simulink model "L1_1"  (R2017b)
settings: Solver=ode4  StartTime=0.0  StopTime=30  FixedStep=0.01  RelTol=1e-3
settings Model: Creator=tutuc  LastModifiedBy=tutuc

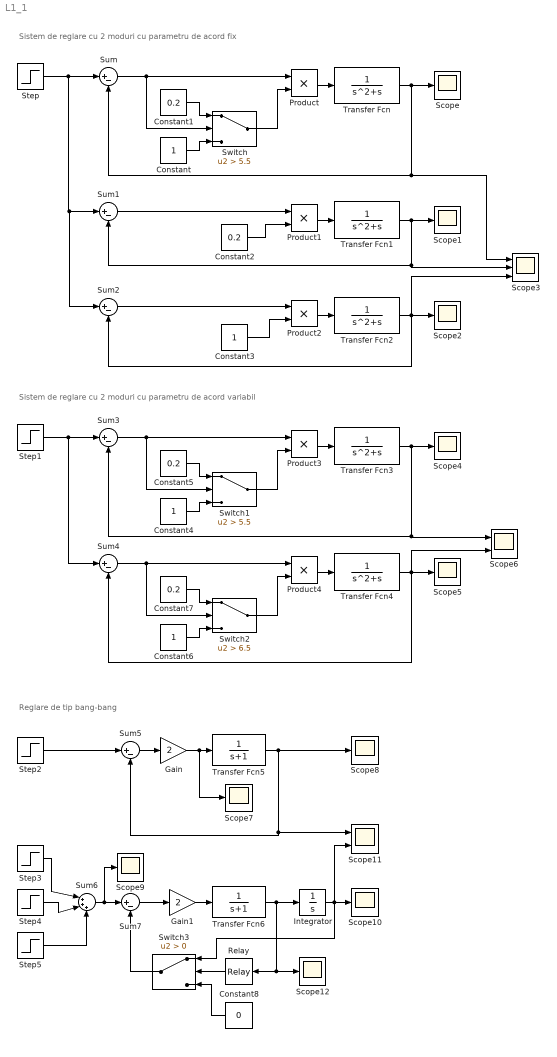
== system L1_1 ==
  note: Sistem de reglare cu 2 moduri cu parametru de acord fix
  note: Sistem de reglare cu 2 moduri cu parametru de acord variabil
  note: Reglare de tip bang-bang
  Constant{,3..4,6} (4 alike) : Constant
  Constant{1..2,5,7} (4 alike) : Constant  Value=0.2
  Constant8 : Constant  Value=0
  Gain : Gain  Gain=2
  Gain1 : Gain  Gain=2
  Integrator : Integrator
  Product{,1..4} (5 alike) : Product
  Relay : Relay  OnSwitchValue=3.1032  OffSwitchValue=-3.1032
  Scope{,1..2,4..5,7..10,12} (10 alike) : Scope
  Scope11 : Scope  NumInputPorts=2
  Scope3 : Scope  NumInputPorts=3
  Scope6 : Scope  NumInputPorts=2
  Step{,1..3} (4 alike) : Step  Time=0  After=10  SampleTime=0
  Step4 : Step  Time=1.35  After=-15  SampleTime=0
  Step5 : Step  Time=1.5  After=5  SampleTime=0
  Sum{,1..5,7} (7 alike) : Sum  Inputs=|+-
  Sum6 : Sum  Inputs=|+++
  Switch : Switch  Criteria=u2 > Threshold  Threshold=5.5
  Switch1 : Switch  Criteria=u2 > Threshold  Threshold=5.5
  Switch2 : Switch  Criteria=u2 > Threshold  Threshold=6.5
  Switch3 : Switch  Criteria=u2 > Threshold
  Transfer Fcn{,1..4} (5 alike) : TransferFcn  Denominator=[1 1 0]
  Transfer Fcn5 : TransferFcn  Denominator=[1 1]
  Transfer Fcn6 : TransferFcn  Denominator=[1 1]
  wires:
  Sum/1 -> Switch/2, Product/1
  Switch/1 -> Product/2
  Step/1 -> Sum2/1, Sum1/1, Sum/1
  Product/1 -> Transfer Fcn/1
  Transfer Fcn/1 -> Scope/1, Sum/2, Scope3/1
  Sum1/1 -> Product1/1
  Constant2/1 -> Product1/2
  Product1/1 -> Transfer Fcn1/1
  Transfer Fcn1/1 -> Scope1/1, Scope3/2, Sum1/2
  Sum2/1 -> Product2/1
  Constant3/1 -> Product2/2
  Product2/1 -> Transfer Fcn2/1
  Transfer Fcn2/1 -> Scope3/3, Scope2/1, Sum2/2
  Constant1/1 -> Switch/1
  Constant/1 -> Switch/3
  Constant4/1 -> Switch1/3
  Constant5/1 -> Switch1/1
  Transfer Fcn3/1 -> Scope6/1, Sum3/2, Scope4/1
  Product3/1 -> Transfer Fcn3/1
  Switch1/1 -> Product3/2
  Sum3/1 -> Product3/1, Switch1/2
  Sum4/1 -> Switch2/2, Product4/1
  Switch2/1 -> Product4/2
  Step1/1 -> Sum3/1, Sum4/1
  Product4/1 -> Transfer Fcn4/1
  Transfer Fcn4/1 -> Scope6/2, Scope5/1, Sum4/2
  Constant7/1 -> Switch2/1
  Constant6/1 -> Switch2/3
  Relay/1 -> Switch3/2
  Gain/1 -> Scope7/1, Transfer Fcn5/1
  Sum7/1 -> Gain1/1
  Switch3/1 -> Sum7/2
  Constant8/1 -> Switch3/3
  Transfer Fcn6/1 -> Scope12/1, Relay/1, Integrator/1
  Step2/1 -> Sum5/1
  Gain1/1 -> Transfer Fcn6/1
  Sum5/1 -> Gain/1
  Step5/1 -> Sum6/3
  Step4/1 -> Sum6/2
  Integrator/1 -> Switch3/1, Scope11/2, Scope10/1
  Step3/1 -> Sum6/1
  Transfer Fcn5/1 -> Sum5/2, Scope11/1, Scope8/1
  Sum6/1 -> Scope9/1, Sum7/1
